simulink model "SIM_model_backup"  (R2026a)
settings: Solver=VariableStepAuto  StopTime=10
libraries: aerolibanim x2, simulink_extras x1
settings Model: Creator=carlos  LastModifiedBy=carlos

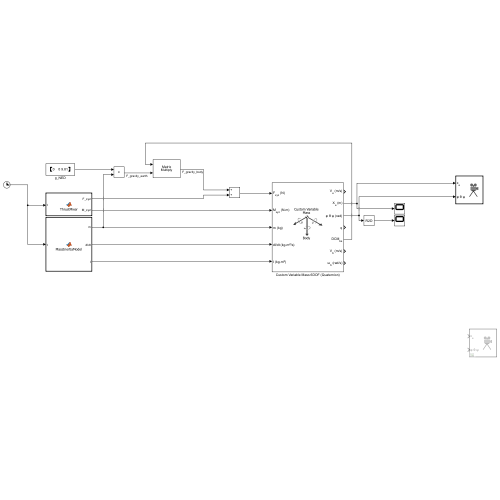
[thumbnail: Simulink's stored preview of the top-level diagram]
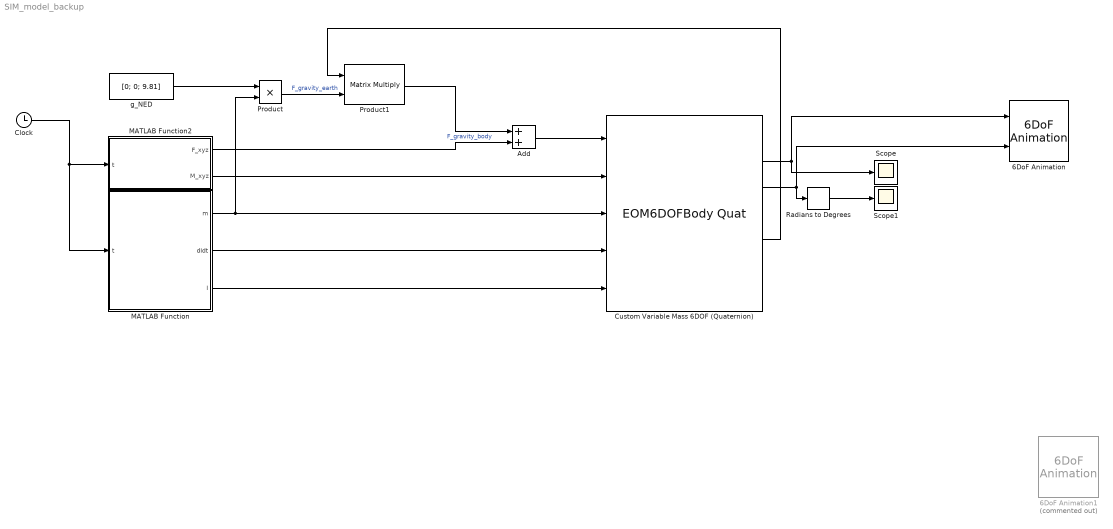
== system SIM_model_backup ==
  6DoF Animation : aerolibanim/6DoF Animation  u1=[-100 100 -100 100 0 3000]  u2=0.1  u3=200  u4=[0 0 0]  u5=Fixed position  u6=[7500 7500 -3150]  u7=10  u8=on
  6DoF Animation1 : aerolibanim/6DoF Animation  Commented=on  u1=[0 4000 -2000 2000 -5000 -3000]  u2=0.1  u3=1.0  u4=[4000 0 -5000]  u5=Fixed position  u6=[2000 500 -3150]  u7=10  u8=on
  Add : Sum
  Clock : Clock
  Custom Variable Mass 6DOF (Quaternion) : EOM6DOFBodyQuat  mtype=Custom Variable  eul_0=[0 deg2rad(90) 0]
  MATLAB Function : MATLAB Function  TreatAsAtomicUnit=on
  MATLAB Function2 : MATLAB Function  TreatAsAtomicUnit=on
  Product : Product
  Product1 : Product  Multiplication=Matrix(*)
  Radians to Degrees : simulink_extras/Transformations/Radians to Degrees
  Scope : Scope
      settings: ActiveDisplayYMinimum=-1052.2268345363707  ActiveDisplayYMaximum=116.91409272630159
  Scope1 : Scope
      settings: ActiveDisplayYMinimum=48.802324300411854  ActiveDisplayYMaximum=194.57751952217646
  g_NED : Constant  Value=[0; 0; 9.81]
  wires:
  MATLAB Function/1(m) -> Product/2, Custom Variable Mass 6DOF (Quaternion)/3
  MATLAB Function/2(dIdt) -> Custom Variable Mass 6DOF (Quaternion)/4
  MATLAB Function/3(I) -> Custom Variable Mass 6DOF (Quaternion)/5
  Clock/1 -> MATLAB Function/1(t), MATLAB Function2/1(t)
  MATLAB Function2/2(M_xyz) -> Custom Variable Mass 6DOF (Quaternion)/2
  g_NED/1 -> Product/1
  Product/1 -> Product1/2  "F_gravity_earth"
  Custom Variable Mass 6DOF (Quaternion)/5 -> Product1/1
  Product1/1 -> Add/1  "F_gravity_body"
  Custom Variable Mass 6DOF (Quaternion)/2 -> Scope/1, 6DoF Animation/1
  Radians to Degrees/1 -> Scope1/1
  Custom Variable Mass 6DOF (Quaternion)/3 -> Radians to Degrees/1, 6DoF Animation/2
  MATLAB Function2/1(F_xyz) -> Add/2
  Add/1 -> Custom Variable Mass 6DOF (Quaternion)/1

== matlab function SIM_model_backup/MATLAB Function2 ==
  data: t input; F_xyz output; M_xyz output
function [F_xyz, M_xyz] = ThrustMixer(t)
% Computes net thrust force and moment from 3 fixed motors
% No gimbal deflection yet - motors point straight along +x_b (nose direction)
% Pure function: no persistent state, safe for continuous solvers

%% --- Editable parameters ---
T_nominal = 8     % N, thrust per motor
t_burn    = 20;      % s, burn duration
r_motor   = 0.10;    % m, radial distance from motor to body x-axis (roll axis)

%% --- Thrust per motor (identical, no variation for now) ---
if t < t_burn
    T = T_nominal * ones(3,1);
else
    T = zeros(3,1);
end

%% --- Motor positions, 120 degrees apart, around the x_b (roll) axis ---
% Motors sit in the y_b - z_b plane (perpendicular to the nose axis)
theta = [0; 120; 240] * pi/180;
r_vec = [zeros(3,1), r_motor*cos(theta), r_motor*sin(theta)];
% each row of r_vec is [rx, ry, rz] for motor k -> rx = 0 (purely radial offset)

%% --- Net force (all thrust along +x_b, no gimbal yet) ---
F_xyz = [sum(T); 0; 0];

%% --- Net moment via cross product r x F, per motor ---
M_xyz = [0; 0; 0];
for k = 1:3
    F_k = [T(k); 0; 0];              % thrust vector of motor k, along +x_b
    M_xyz = M_xyz + cross(r_vec(k,:)', F_k);
end

end

== matlab function SIM_model_backup/MATLAB Function ==
  data: t input; m output; dIdt output; I output
function [m, dIdt, I] = MassInertiaModel(t)
% Computes vehicle mass and inertia tensor as propellant burns
% Linear depletion model: mass decreases linearly during burn, then holds constant

%% --- Editable parameters ---
m_dry    = 0.8;    % kg, mass with no propellant (structure + avionics + empty motors)
m_prop   = 0.05;   % kg, total propellant mass (KNSB)
t_burn   = 20;     % s, burn duration (must match ThrustMixer)

Ixx_dry  = 0.002;  % kg*m^2, roll-axis inertia (about x_b, nose axis), empty
Iyy_dry  = 0.05;   % kg*m^2, pitch-axis inertia (about y_b), empty
Izz_dry  = 0.05;   % kg*m^2, yaw-axis inertia (about z_b), empty

% How much extra inertia the propellant mass contributes when full
% (rough approximation: propellant sits near the tail, contributes mostly to pitch/yaw)
Ixx_prop = 0.0002;
Iyy_prop = 0.01;
Izz_prop = 0.01;

%% --- Mass as a function of time ---
if t < t_burn
    frac_burned = t / t_burn;      % 0 at ignition, 1 at burnout
else
    frac_burned = 1;
end

m_remaining_prop = m_prop * (1 - frac_burned);
m = m_dry + m_remaining_prop;

%% --- Inertia as a function of remaining propellant ---
Ixx = Ixx_dry + Ixx_prop * (1 - frac_burned);
Iyy = Iyy_dry + Iyy_prop * (1 - frac_burned);
Izz = Izz_dry + Izz_prop * (1 - frac_burned);

I = [Ixx 0 0; 0 Iyy 0; 0 0 Izz];

%% --- dI/dt (derivative of inertia w.r.t. time) ---
if t < t_burn
    dIxx_dt = -Ixx_prop / t_burn;
    dIyy_dt = -Iyy_prop / t_burn;
    dIzz_dt = -Izz_prop / t_burn;
else
    dIxx_dt = 0;
    dIyy_dt = 0;
    dIzz_dt = 0;
end

dIdt = [dIxx_dt 0 0; 0 dIyy_dt 0; 0 0 dIzz_dt];

end
